simulink model "Register_File"  (R2021a)
settings: Solver=VariableStepAuto  StartTime=0.0  StopTime=10.0  RelTol=1e-3
libraries: dspsigops x4
settings Model: Creator=kbhar  LastModifiedBy=kbhar

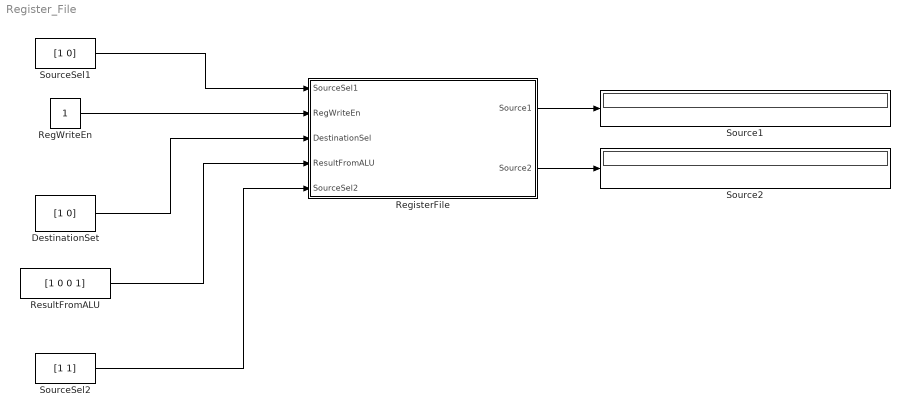
== system Register_File ==
  DestinationSet : Constant  Value=[1 0]
  RegWriteEn : Constant
  RegisterFile : Subsystem
  ResultFromALU : Constant  Value=[1 0 0 1]
  Source1 : Display
  Source2 : Display
  SourceSel1 : Constant  Value=[1 0]
  SourceSel2 : Constant  Value=[1 1]
  wires:
  SourceSel1/1 -> RegisterFile/1(SourceSel1)
  RegWriteEn/1 -> RegisterFile/2(RegWriteEn)
  DestinationSet/1 -> RegisterFile/3(DestinationSel)
  ResultFromALU/1 -> RegisterFile/4(ResultFromALU)
  SourceSel2/1 -> RegisterFile/5(SourceSel2)
  RegisterFile/1(Source1) -> Source1/1
  RegisterFile/2(Source2) -> Source2/1

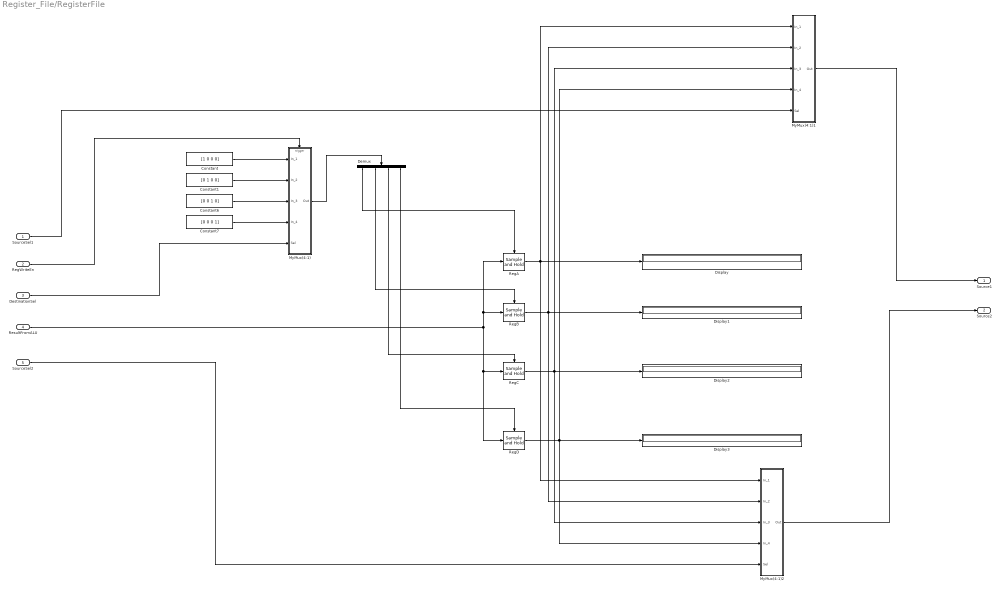
== system Register_File/RegisterFile ==
  SourceSel1 : Inport
  RegWriteEn : Inport  Port=2
  DestinationSel : Inport  Port=3
  ResultFromALU : Inport  Port=4
  SourceSel2 : Inport  Port=5
  Constant : Constant  Value=[1 0 0 0]
  Constant1 : Constant  Value=[0 1 0 0]
  Constant6 : Constant  Value=[0 0 1 0]
  Constant7 : Constant  Value=[0 0 0 1]
  Demux : Demux
  Display{,1..3} (4 alike) : Display
  MyMux(4:1) : Subsystem
  MyMux(4:1)1 : Subsystem
  MyMux(4:1)2 : Subsystem
  RegA : dspsigops/Sample and Hold  trig=Rising edge  initCond=[1 0 0 0]  latchinput=off
  RegB : dspsigops/Sample and Hold  trig=Rising edge  initCond=[0 1 0 0]  latchinput=off
  RegC : dspsigops/Sample and Hold  trig=Rising edge  initCond=[0 1 0 1]  latchinput=off
  RegD : dspsigops/Sample and Hold  trig=Rising edge  initCond=[0 0 0 1]  latchinput=off
  Source1 : Outport
  Source2 : Outport  Port=2
  wires:
  ResultFromALU/1 -> RegD/1, RegC/1, RegA/1, RegB/1
  RegB/1 -> MyMux(4:1)2/2(In_2), MyMux(4:1)1/2(In_2), Display1/1
  RegC/1 -> MyMux(4:1)2/3(In_3), MyMux(4:1)1/3(In_3), Display2/1
  Demux/1 -> RegA/Trigger
  RegA/1 -> MyMux(4:1)2/1(In_1), MyMux(4:1)1/1(In_1), Display/1
  Constant7/1 -> MyMux(4:1)/4(In_4)
  RegD/1 -> MyMux(4:1)2/4(In_4), MyMux(4:1)1/4(In_4), Display3/1
  Constant/1 -> MyMux(4:1)/1(In_1)
  Constant6/1 -> MyMux(4:1)/3(In_3)
  Constant1/1 -> MyMux(4:1)/2(In_2)
  Demux/4 -> RegD/Trigger
  SourceSel1/1 -> MyMux(4:1)1/5(Sel)
  Demux/3 -> RegC/Trigger
  MyMux(4:1)1/1(Out) -> Source1/1
  Demux/2 -> RegB/Trigger
  DestinationSel/1 -> MyMux(4:1)/5(Sel)
  MyMux(4:1)/1(Out) -> Demux/1
  RegWriteEn/1 -> MyMux(4:1)/Trigger
  SourceSel2/1 -> MyMux(4:1)2/5(Sel)
  MyMux(4:1)2/1(Out) -> Source2/1

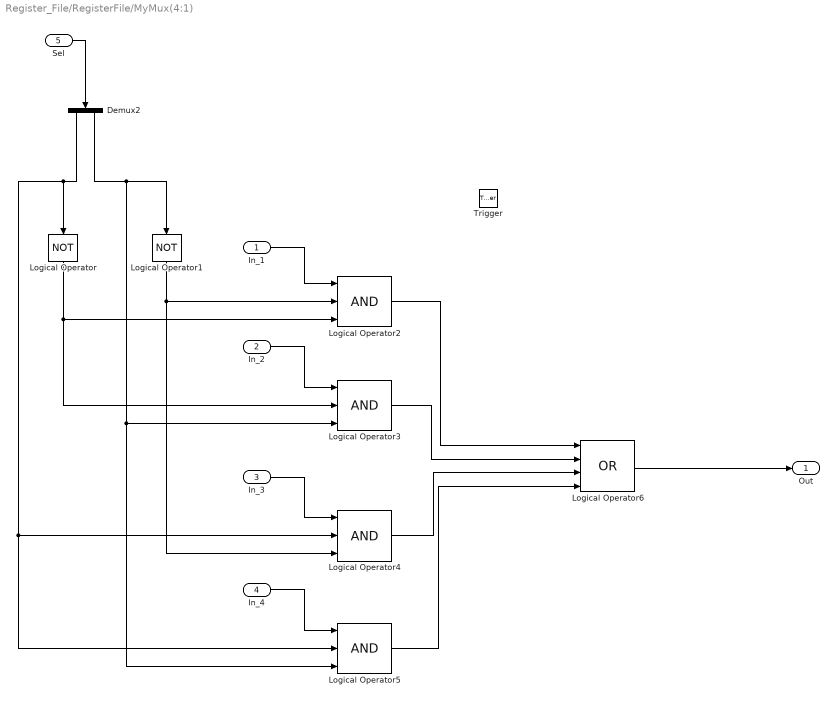
== system Register_File/RegisterFile/MyMux(4:1) ==
  In_1 : Inport
  In_2 : Inport  Port=2
  In_3 : Inport  Port=3
  In_4 : Inport  Port=4
  Sel : Inport  Port=5
  Trigger : TriggerPort  VariantControl=(inherit)  PortDimensions=1
  Demux2 : Demux  Outputs=2
  Logical Operator : Logic  Operator=NOT  AllPortsSameDT=off  OutDataTypeStr=boolean
  Logical Operator1 : Logic  Operator=NOT  AllPortsSameDT=off  OutDataTypeStr=boolean
  Logical Operator{2..5} (4 alike) : Logic  Inputs=3  AllPortsSameDT=off  OutDataTypeStr=boolean
  Logical Operator6 : Logic  Operator=OR  Inputs=4  AllPortsSameDT=off  OutDataTypeStr=boolean
  Out : Outport
  wires:
  Demux2/1 -> Logical Operator4/2, Logical Operator5/2, Logical Operator/1
  Demux2/2 -> Logical Operator5/3, Logical Operator3/3, Logical Operator1/1
  Logical Operator1/1 -> Logical Operator2/2, Logical Operator4/3
  Logical Operator2/1 -> Logical Operator6/1
  Logical Operator3/1 -> Logical Operator6/2
  Logical Operator/1 -> Logical Operator2/3, Logical Operator3/2
  Logical Operator4/1 -> Logical Operator6/3
  Logical Operator5/1 -> Logical Operator6/4
  In_2/1 -> Logical Operator3/1
  In_3/1 -> Logical Operator4/1
  In_4/1 -> Logical Operator5/1
  In_1/1 -> Logical Operator2/1
  Logical Operator6/1 -> Out/1
  Sel/1 -> Demux2/1

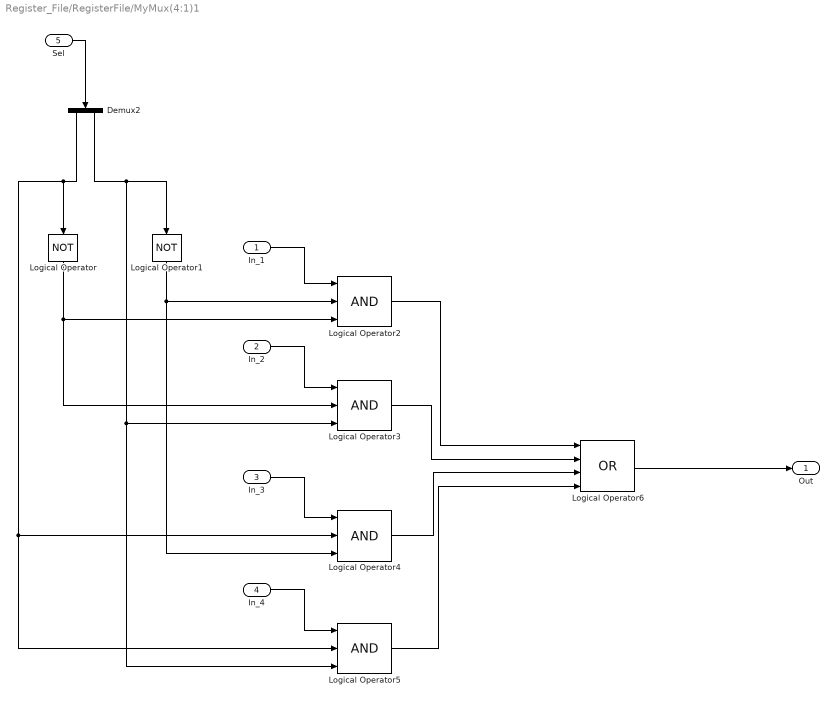
== system Register_File/RegisterFile/MyMux(4:1)1 ==
  In_1 : Inport
  In_2 : Inport  Port=2
  In_3 : Inport  Port=3
  In_4 : Inport  Port=4
  Sel : Inport  Port=5
  Demux2 : Demux  Outputs=2
  Logical Operator : Logic  Operator=NOT  AllPortsSameDT=off  OutDataTypeStr=boolean
  Logical Operator1 : Logic  Operator=NOT  AllPortsSameDT=off  OutDataTypeStr=boolean
  Logical Operator{2..5} (4 alike) : Logic  Inputs=3  AllPortsSameDT=off  OutDataTypeStr=boolean
  Logical Operator6 : Logic  Operator=OR  Inputs=4  AllPortsSameDT=off  OutDataTypeStr=boolean
  Out : Outport
  wires:
  Demux2/1 -> Logical Operator4/2, Logical Operator5/2, Logical Operator/1
  Demux2/2 -> Logical Operator5/3, Logical Operator3/3, Logical Operator1/1
  Logical Operator1/1 -> Logical Operator2/2, Logical Operator4/3
  Logical Operator2/1 -> Logical Operator6/1
  Logical Operator3/1 -> Logical Operator6/2
  Logical Operator/1 -> Logical Operator2/3, Logical Operator3/2
  Logical Operator4/1 -> Logical Operator6/3
  Logical Operator5/1 -> Logical Operator6/4
  In_2/1 -> Logical Operator3/1
  In_3/1 -> Logical Operator4/1
  In_4/1 -> Logical Operator5/1
  In_1/1 -> Logical Operator2/1
  Logical Operator6/1 -> Out/1
  Sel/1 -> Demux2/1

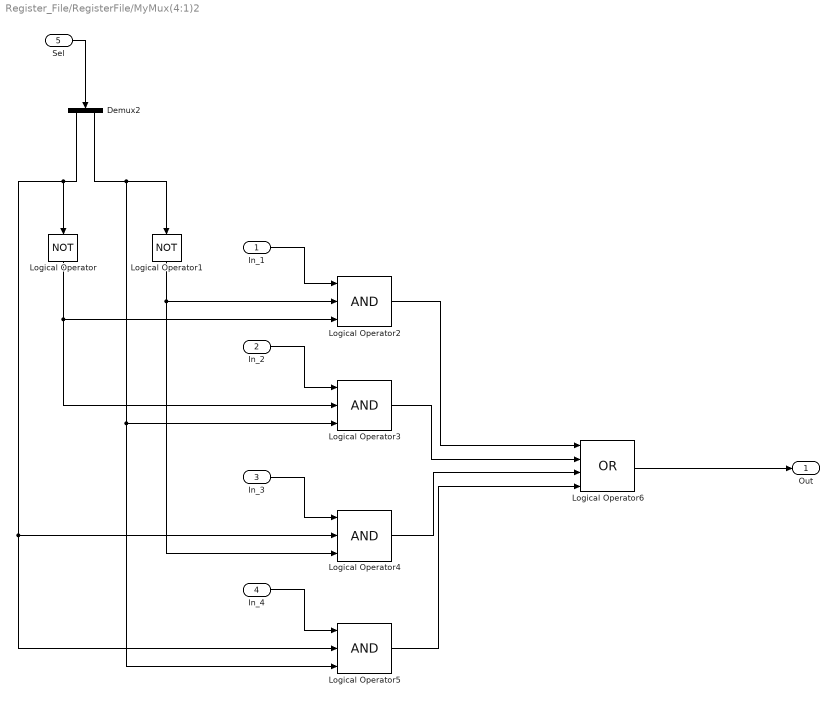
== system Register_File/RegisterFile/MyMux(4:1)2 ==
  In_1 : Inport
  In_2 : Inport  Port=2
  In_3 : Inport  Port=3
  In_4 : Inport  Port=4
  Sel : Inport  Port=5
  Demux2 : Demux  Outputs=2
  Logical Operator : Logic  Operator=NOT  AllPortsSameDT=off  OutDataTypeStr=boolean
  Logical Operator1 : Logic  Operator=NOT  AllPortsSameDT=off  OutDataTypeStr=boolean
  Logical Operator{2..5} (4 alike) : Logic  Inputs=3  AllPortsSameDT=off  OutDataTypeStr=boolean
  Logical Operator6 : Logic  Operator=OR  Inputs=4  AllPortsSameDT=off  OutDataTypeStr=boolean
  Out : Outport
  wires:
  Demux2/1 -> Logical Operator4/2, Logical Operator5/2, Logical Operator/1
  Demux2/2 -> Logical Operator5/3, Logical Operator3/3, Logical Operator1/1
  Logical Operator1/1 -> Logical Operator2/2, Logical Operator4/3
  Logical Operator2/1 -> Logical Operator6/1
  Logical Operator3/1 -> Logical Operator6/2
  Logical Operator/1 -> Logical Operator2/3, Logical Operator3/2
  Logical Operator4/1 -> Logical Operator6/3
  Logical Operator5/1 -> Logical Operator6/4
  In_2/1 -> Logical Operator3/1
  In_3/1 -> Logical Operator4/1
  In_4/1 -> Logical Operator5/1
  In_1/1 -> Logical Operator2/1
  Logical Operator6/1 -> Out/1
  Sel/1 -> Demux2/1
